simulink model "udp_test"  (R2022b)
settings: Solver=FixedStepAuto  StartTime=0.0  StopTime=100  FixedStep=Ts  RelTol=1e-3
InitFcn:
  | Ts = 1e-5;
undefined symbols (not defined in the file): f
libraries: slrealtimeutilitieslib x2, slrealtimeiplib x2, instrumentlib x2
settings Model: Creator=Javnson  LastModifiedBy=Javnson

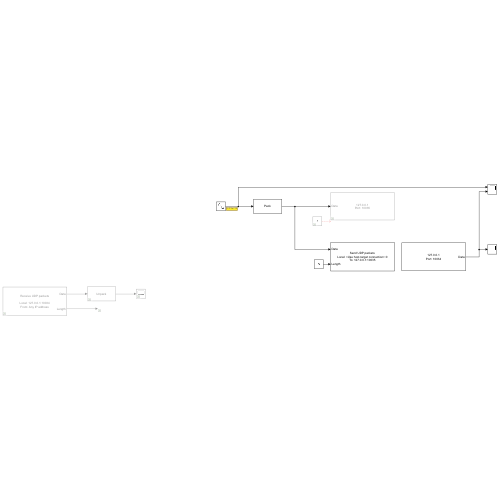
[thumbnail: Simulink's stored preview of the top-level diagram]
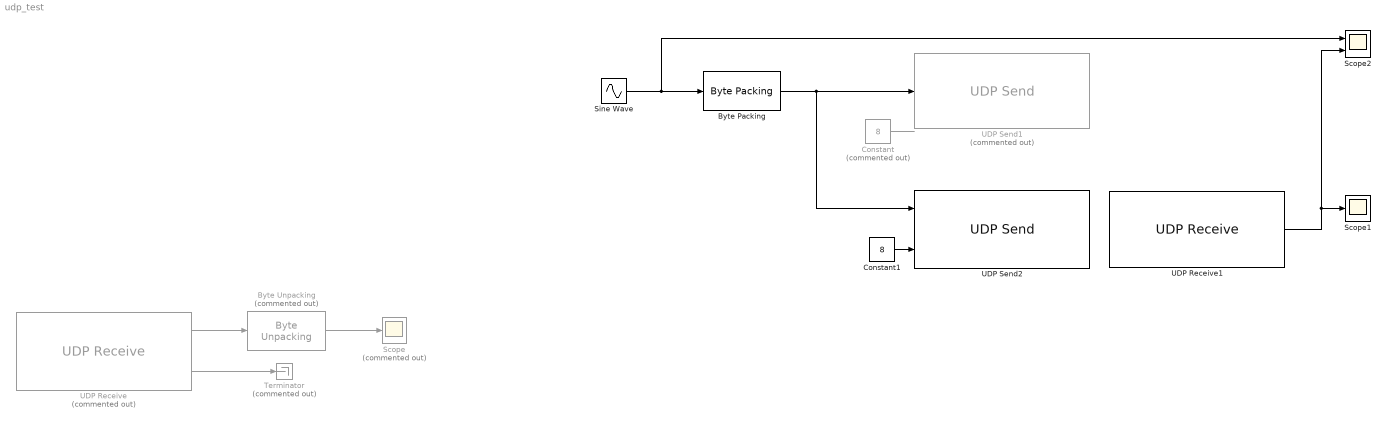
== system udp_test ==
  Byte Packing : slrealtimeutilitieslib/Byte Packing  MaskPackedDataType=uint8  MaskUnpackedDataTypes={'double'}  MaskAlignment=1
  Byte Unpacking : slrealtimeutilitieslib/Byte Unpacking  Commented=on  MaskUnpackedDataTypes={'double'}  MaskUnpackedDataSizes={[1]}  MaskAlignment=1
  Constant : Constant  Commented=on  Value=8
  Constant1 : Constant  Value=8
  Scope : Scope  Commented=on
  Scope1 : Scope
  Scope2 : Scope  NumInputPorts=2
  Sine Wave : Sin  Frequency=pi*10  SampleTime=Ts
  Terminator : Terminator  Commented=on
  UDP Receive : slrealtimeiplib/UDP Receive  Commented=on  useHostTargetConn=off  ipAddress=127.0.0.1  localPort=10034  rcvWidth=8  rcvFmAny=on  fmAddress='10.10.10.10'  sampleTime=-1  enableMessage=off  maxPackets=1
  UDP Receive1 : instrumentlib/UDP Receive  LocalAddress=127.0.0.1  LocalPort=10034  EnablePortSharing=off  Host=localhost  Port=10034  GetLatestData=on  DataSize=[ 1 ]  DataType=double  ASCIIFormatting=%f,  Terminator=LF  CustomTerminator=10  ByteOrder=little-endian  EnableBlockingMode=on  Timeout=20  SampleTime=0.01  SimulateUsing=Interpreted execution
  UDP Send1 : instrumentlib/UDP Send  Commented=on  Host=127.0.0.1  Port=10035  LocalAddress=0.0.0.0  LocalPort=10035  EnablePortSharing=on  OutputDatagramPacketSize=8  ByteOrder=big-endian  EnableBlockingMode=on  SimulateUsing=Interpreted execution
  UDP Send2 : slrealtimeiplib/UDP Send  useHostTargetConn=on  toAddress='127.0.0.1'  toPort=10035  sampleTime=0.01  enableMessage=off
  wires:
  Byte Unpacking/1 -> Scope/1
  UDP Receive/2 -> Terminator/1
  UDP Receive/1 -> Byte Unpacking/1
  UDP Receive1/1 -> Scope2/2, Scope1/1
  Sine Wave/1 -> Scope2/1, Byte Packing/1
  Byte Packing/1 -> UDP Send1/1, UDP Send2/1
  Constant/1 -> ?
  Constant1/1 -> UDP Send2/2
